simulink model "ctrl_PF"  (R2022b)
settings: Solver=FixedStepAuto  StartTime=0.0  StopTime=Tf  FixedStep=0.05  RelTol=1e-3
StopFcn:
  | save('testdata')
values from neighbouring files (symbols this model uses):
  Ba_0 = [0 0 0 0 0 0]    [run.m]    (also in testdata.mat)
  Bb = 4418825.3321    [testdata.mat]
  Bv_0 = [-5.14444 0 0 0 0 0]    [run.m]    (also in testdata.mat)
  Bx_0 = [-Cp(1,1) -Cp(2,1) Cp(3,1) 0 0 -pi]    [run.m]    (also in testdata.mat = [7.34788079488e-14 -400 -100 0 0 -3.14159265359])
  Cp = [x;y;z]    [run.m]    (also in testdata.mat = [-7.34788079488e-14 400 -100 -24.1026674607 399.273166418 -1)
  Cp_prime = Cp*Diff    [run.m]    (also in testdata.mat = [-4.77232815721 -0.143913049279 0 -4.75515990164 -0.42831409)
  d = 50    [run.m]    (also in testdata.mat)
  dA_BP1 = [0.00388591051125 0.00354364911083 0.00553040741788 0.00502167988714 0.0078585088908 0.00748424955325 0.0119232766011 0.0109054787122 0.0168329706434 0.016985509009 0.0156802934897 0.014556760782 ... (616 elements, 616x1)]    [testdata.mat]
  dA_BP2 = [0.00388594063171 0.00354357191533 0.00553040491113 0.00502170939051 0.00785855989083 0.00748435285791 0.0119232653011 0.0109054419481 0.0168329955973 0.0169854794658 0.015680230324 0.0145567225609 ... (616 elements, 616x1)]    [testdata.mat]
  dA_Hull = [0.896301676511 0.898896720864 0.884294141897 0.886832830172 0.870887902011 0.873360353662 0.856223658523 0.858613244346 0.840314828191 0.842595287849 0.823129385532 0.8253007603 ... (2914 elements, 2914x1)]    [testdata.mat]
  dA_PH = [0.00917454029683 0.00917454029683 0.00646521761836 0.00644666811643 0.011728531678 0.0107683420972 0.0165186720105 0.0100399866209 0.0121147162203 0.00917369783051 0.00917369783051 0.00646462373197 ... (550 elements, 550x1)]    [testdata.mat]
  dA_Sail = [0.08073747293 0.0655437895785 0.0678199581962 0.211496702297 0.185444652254 0.10949647106 0.0763960001413 0.0735864235671 0.0440728222699 0.281106392154 0.32735958292 0.104041938486 ... (564 elements, 564x1)]    [testdata.mat]
  dA_SProot = [0.0225345452169 0.0247277274893 0.0225345452169 0.0480467976325 0.0166447079844 0.0410754287554 0.0247277274893 0.0480467976325 0.0468898715351 0.0839833312794 0.0166447079844 0.0255016718 ... (904 elements, 904x1)]    [testdata.mat]
  dA_X1a = [0.0149621011817 0.0166706156701 0.0341149781095 0.0355915100668 0.0512235531199 0.0489176133683 0.0604458424392 0.0503279152264 0.0577124835488 0.0401555322121 0.044833653096 0.0251568218541 ... (200 elements, 200x1)]    [testdata.mat]
  dA_X1b = [0.0149621011817 0.0166706156701 0.0341149781095 0.0355915100668 0.0512235531199 0.0489176133683 0.0604458424392 0.0503279152264 0.0577124835488 0.0401555322121 0.044833653096 0.0251568218541 ... (200 elements, 200x1)]    [testdata.mat]
  dA_X2a = [0.0149620639393 0.0166705502855 0.0341150948266 0.0355913495849 0.051223110376 0.0489180393921 0.0604458270347 0.0503275686692 0.0577128112225 0.0401556683139 0.0448334591683 0.0251566482124 ... (200 elements, 200x1)]    [testdata.mat]
  dA_X2b = [0.0149620639393 0.0166705502855 0.0341150948266 0.0355913495849 0.051223110376 0.0489180393921 0.0604458270347 0.0503275686692 0.0577128112225 0.0401556683139 0.0448334591683 0.0251566482124 ... (200 elements, 200x1)]    [testdata.mat]
  dA_X3a = [0.0149621011817 0.0166706156701 0.0341149781095 0.0355915100668 0.0512235531199 0.0489176133683 0.0604458424392 0.0503279152264 0.0577124835488 0.0401555322121 0.044833653096 0.0251568218541 ... (200 elements, 200x1)]    [testdata.mat]
  dA_X3b = [0.0149621011817 0.0166706156701 0.0341149781095 0.0355915100668 0.0512235531199 0.0489176133683 0.0604458424392 0.0503279152264 0.0577124835488 0.0401555322121 0.044833653096 0.0251568218541 ... (200 elements, 200x1)]    [testdata.mat]
  dA_X4a = [0.0149621011817 0.0166706156701 0.0341149781095 0.0355915100668 0.0512235531199 0.0489176133683 0.0604458424392 0.0503279152264 0.0577124835488 0.0401555322121 0.044833653096 0.0251568218541 ... (200 elements, 200x1)]    [testdata.mat]
  dA_X4b = [0.0149621011817 0.0166706156701 0.0341149781095 0.0355915100668 0.0512235531199 0.0489176133683 0.0604458424392 0.0503279152264 0.0577124835488 0.0401555322121 0.044833653096 0.0251568218541 ... (200 elements, 200x1)]    [testdata.mat]
  Ixx = 52300000    [testdata.mat]
  Ixy = 0    [testdata.mat]
  Ixz = 0    [testdata.mat]
  Iyy = 1375000000    [testdata.mat]
  Iyz = 0    [testdata.mat]
  Izz = 1367000000    [testdata.mat]
  Ky = 1    [run.m]    (also in testdata.mat)
  Mb = 4418825.3321    [testdata.mat]
  n_BP1 = [-0.7747315 -0.03638153 -0.4095958 0 -0.1221389 0 -0.01670914 0 0.005209626 0 0.03404154 0 ... (1848 elements, 616x3)]    [testdata.mat]
  n_BP2 = [-0.774731517 -0.0363815315 -0.409595788 0 -0.122138903 0 -0.0167091396 0 0.00520962616 0 0.0340415388 0 ... (1848 elements, 616x3)]    [testdata.mat]
  n_Hull = [-3.334458e-05 -1.700098e-14 -3.354233e-05 -1.686235e-14 -3.289162e-05 -1.685701e-14 -3.291391e-05 -1.698144e-14 -3.338145e-05 -1.688959e-14 -3.29289e-05 -1.682536e-14 ... (8742 elements, 2914x3)]    [testdata.mat]
  n_PH = [0 0 0.01711651 0.01711627 0.2676807 0.2676804 0.7675173 0.7675174 0.9857236 0 0 0.01711456 ... (1650 elements, 550x3)]    [testdata.mat]
  n_Sail = [-0.05126832 -0.05168081 -0.0485872 -0.03288998 -0.03203588 -0.04435105 -0.04335441 -0.04419429 -0.05169604 0.01094904 0.01649325 -0.03825178 ... (1692 elements, 564x3)]    [testdata.mat]
  n_SProot = [-0.7837688 -0.7969784 -0.7837688 -0.79448 -0.280412 -0.3378876 -0.7969784 -0.79448 -0.7910827 -0.3483897 -0.280412 -0.2790298 ... (2712 elements, 904x3)]    [testdata.mat]
  n_X2a = [-0.283297986 -0.283136904 -0.283195704 -0.28313759 -0.2831586 -0.283137113 -0.28313911 -0.283136606 -0.283121586 -0.283136815 -0.283108413 -0.283138901 ... (600 elements, 200x3)]    [testdata.mat]
  n_X2b = [-0.283297986 -0.283136904 -0.283195704 -0.28313759 -0.2831586 -0.283137113 -0.28313911 -0.283136606 -0.283121586 -0.283136815 -0.283108413 -0.283138901 ... (600 elements, 200x3)]    [testdata.mat]
  n_X3a = [-0.283298 -0.2831369 -0.2831957 -0.2831376 -0.2831586 -0.2831371 -0.2831391 -0.2831366 -0.2831216 -0.2831368 -0.2831084 -0.2831389 ... (600 elements, 200x3)]    [testdata.mat]
  n_X4a = [-0.283298 -0.2831369 -0.2831957 -0.2831376 -0.2831586 -0.2831371 -0.2831391 -0.2831366 -0.2831216 -0.2831368 -0.2831084 -0.2831389 ... (600 elements, 200x3)]    [testdata.mat]
  n_X4b = [-0.283298 -0.2831369 -0.2831957 -0.2831376 -0.2831586 -0.2831371 -0.2831391 -0.2831366 -0.2831216 -0.2831368 -0.2831084 -0.2831389 ... (600 elements, 200x3)]    [testdata.mat]
  nt_BP1 = 616    [testdata.mat]
  nt_BP2 = 616    [testdata.mat]
  nt_Hull = 2914    [testdata.mat]
  nt_PH = 550    [testdata.mat]
  nt_Sail = 564    [testdata.mat]
  nt_SProot = 904    [testdata.mat]
  nt_X1a = 200    [testdata.mat]
  nt_X1b = 200    [testdata.mat]
  nt_X2a = 200    [testdata.mat]
  nt_X2b = 200    [testdata.mat]
  nt_X3a = 200    [testdata.mat]
  nt_X3b = 200    [testdata.mat]
  nt_X4a = 200    [testdata.mat]
  nt_X4b = 200    [testdata.mat]
  Seastate = 0    [run.m]    (also in testdata.mat)
  Tf = 500    [run.m]    (also in testdata.mat)
  v_ref = Bv_0(1)    [run.m]    (also in testdata.mat = -5.14444)
  vt1_BP1 = [-11.0524049722 -10.9924120522 -10.9924120522 -10.8819663922 -10.8819663922 -10.7297166322 -10.7297166322 -10.5070632922 -10.5070632922 -10.1807245522 -10.1807245522 -9.8815181122 ... (1848 elements, 616x3)]    [testdata.mat]
  vt1_BP2 = [-11.0524048318 -10.9924111396 -10.9924111396 -10.8819658306 -10.8819658306 -10.7297157898 -10.7297157898 -10.5070637134 -10.5070637134 -10.1807238502 -10.1807238502 -9.8815188844 ... (1848 elements, 616x3)]    [testdata.mat]
  vt1_Hull = [3.5122487678 3.7304022878 5.2621803278 5.4863499878 6.9866994878 7.2167238278 8.6832650078 8.9189474678 10.3493567078 10.5904445678 11.9823842078 12.2286247478 ... (8742 elements, 2914x3)]    [testdata.mat]
  vt1_PH = [37.3342788278 37.3342788278 37.4268866678 37.4268866678 37.5892452278 37.5892452278 37.7549453078 37.7549453078 37.8074619278 37.3342788278 37.3342788278 37.4268866678 ... (1650 elements, 550x3)]    [testdata.mat]
  vt1_Sail = [-12.4909433722 -12.1578443722 -12.0399645322 -11.2138368922 -10.6240515922 -11.5111900522 -11.9364967522 -11.6561249722 -12.4909433722 -7.5732648922 -6.8453119522 -11.1890071522 ... (1692 elements, 564x3)]    [testdata.mat]
  vt1_SProot = [29.2099766678 29.1371231078 29.0494854278 29.2099766678 29.2862630078 29.4526510478 29.0494854278 29.1261368078 29.3369263478 29.5706712878 29.0494854278 29.3857364078 ... (2712 elements, 904x3)]    [testdata.mat]
  vt1_X1a = [29.3961751478 29.4776282078 29.4776282078 29.7060309278 29.7060309278 30.0693861278 30.0693861278 30.5458756478 30.5458756478 31.0830460478 31.0830460478 31.6023926678 ... (600 elements, 200x3)]    [testdata.mat]
  vt1_X1b = [29.6638337078 29.6638337078 29.9620713878 29.9620713878 30.3181187678 30.3181187678 30.7116389078 30.7116389078 31.1104380878 31.1104380878 31.4810519678 31.4810519678 ... (600 elements, 200x3)]    [testdata.mat]
  vt1_X2a = [29.3961767624 29.4776272952 29.4776272952 29.7060326828 29.7060326828 30.0693842324 30.0693842324 30.5458736822 30.5458736822 31.083047171 31.083047171 31.6023916148 ... (600 elements, 200x3)]    [testdata.mat]
  vt1_X2b = [29.6638345502 29.6638345502 29.9620708964 29.9620708964 30.3181168022 30.3181168022 30.7116409436 30.7116409436 31.1104372454 31.1104372454 31.4810526698 31.4810526698 ... (600 elements, 200x3)]    [testdata.mat]
  vt1_X3a = [29.3961751478 29.4776282078 29.4776282078 29.7060309278 29.7060309278 30.0693861278 30.0693861278 30.5458756478 30.5458756478 31.0830460478 31.0830460478 31.6023926678 ... (600 elements, 200x3)]    [testdata.mat]
  vt1_X3b = [29.6638337078 29.6638337078 29.9620713878 29.9620713878 30.3181187678 30.3181187678 30.7116389078 30.7116389078 31.1104380878 31.1104380878 31.4810519678 31.4810519678 ... (600 elements, 200x3)]    [testdata.mat]
  vt1_X4a = [29.6638337078 29.6638337078 29.9620713878 29.9620713878 30.3181187678 30.3181187678 30.7116389078 30.7116389078 31.1104380878 31.1104380878 31.4810519678 31.4810519678 ... (600 elements, 200x3)]    [testdata.mat]
  vt1_X4b = [29.3961751478 29.4776282078 29.4776282078 29.7060309278 29.7060309278 30.0693861278 30.0693861278 30.5458756478 30.5458756478 31.0830460478 31.0830460478 31.6023926678 ... (600 elements, 200x3)]    [testdata.mat]
  vt2_BP1 = [-10.9924120522 -10.9494777322 -10.8819663922 -10.8505308322 -10.7297166322 -10.7112259522 -10.5070632922 -10.4997203722 -10.1807245522 -10.1757543922 -9.8815181122 -9.8813004922 ... (1848 elements, 616x3)]    [testdata.mat]
  vt2_BP2 = [-11.0294626294 -11.0294626294 -10.9494786448 -10.9494786448 -10.8505316746 -10.8505316746 -10.7112256012 -10.7112256012 -10.499720302 -10.499720302 -10.1757550942 -10.1757550942 ... (1848 elements, 616x3)]    [testdata.mat]
  vt2_Hull = [1.9517168078 1.9517168078 3.7304022878 3.7304022878 5.4863499878 5.4863499878 7.2167238278 7.2167238278 8.9189474678 8.9189474678 10.5904445678 10.5904445678 ... (8742 elements, 2914x3)]    [testdata.mat]
  vt2_PH = [37.2028433678 37.2028433678 37.3342788278 37.4268866678 37.4268866678 37.5892452278 37.5892452278 37.7549453078 37.7549453078 37.2028433678 37.2028433678 37.3342788278 ... (1650 elements, 550x3)]    [testdata.mat]
  vt2_Sail = [-12.0399645322 -12.0399645322 -11.9364967522 -10.7084881522 -10.7084881522 -12.0399645322 -12.0399645322 -11.9364967522 -12.3734566522 -7.7110323922 -7.7110323922 -11.6561249722 ... (1692 elements, 564x3)]    [testdata.mat]
  vt2_SProot = [29.0494854278 29.0494854278 29.2099766678 29.1261368078 29.0494854278 29.1371231078 29.1371231078 29.2099766678 29.1261368078 29.2099766678 29.2862630078 29.2862630078 ... (2712 elements, 904x3)]    [testdata.mat]
  vt2_X1a = [29.4776282078 29.9620713878 29.7060309278 30.3181187678 30.0693861278 30.7116389078 30.5458756478 31.1104380878 31.0830460478 31.4810519678 31.6023926678 31.7970362078 ... (600 elements, 200x3)]    [testdata.mat]
  vt2_X1b = [29.4776282078 29.9620713878 29.7060309278 30.3181187678 30.0693861278 30.7116389078 30.5458756478 31.1104380878 31.0830460478 31.4810519678 31.6023926678 31.7970362078 ... (600 elements, 200x3)]    [testdata.mat]
  vt2_X2a = [29.6638345502 29.6638345502 29.9620708964 29.9620708964 30.3181168022 30.3181168022 30.7116409436 30.7116409436 31.1104372454 31.1104372454 31.4810526698 31.4810526698 ... (600 elements, 200x3)]    [testdata.mat]
  vt2_X2b = [29.3961767624 29.4776272952 29.4776272952 29.7060326828 29.7060326828 30.0693842324 30.0693842324 30.5458736822 30.5458736822 31.083047171 31.083047171 31.6023916148 ... (600 elements, 200x3)]    [testdata.mat]
  vt2_X3a = [29.4776282078 29.9620713878 29.7060309278 30.3181187678 30.0693861278 30.7116389078 30.5458756478 31.1104380878 31.0830460478 31.4810519678 31.6023926678 31.7970362078 ... (600 elements, 200x3)]    [testdata.mat]
  vt2_X3b = [29.4776282078 29.9620713878 29.7060309278 30.3181187678 30.0693861278 30.7116389078 30.5458756478 31.1104380878 31.0830460478 31.4810519678 31.6023926678 31.7970362078 ... (600 elements, 200x3)]    [testdata.mat]
  vt2_X4a = [29.4776282078 29.9620713878 29.7060309278 30.3181187678 30.0693861278 30.7116389078 30.5458756478 31.1104380878 31.0830460478 31.4810519678 31.6023926678 31.7970362078 ... (600 elements, 200x3)]    [testdata.mat]
  vt2_X4b = [29.4776282078 29.9620713878 29.7060309278 30.3181187678 30.0693861278 30.7116389078 30.5458756478 31.1104380878 31.0830460478 31.4810519678 31.6023926678 31.7970362078 ... (600 elements, 200x3)]    [testdata.mat]
  vt3_BP1 = [-11.0294636122 -11.0294636122 -10.9494777322 -10.9494777322 -10.8505308322 -10.8505308322 -10.7112259522 -10.7112259522 -10.4997203722 -10.4997203722 -10.1757543922 -10.1757543922 ... (1848 elements, 616x3)]    [testdata.mat]
  vt3_BP2 = [-10.9924111396 -10.9494786448 -10.8819658306 -10.8505316746 -10.7297157898 -10.7112256012 -10.5070637134 -10.499720302 -10.1807238502 -10.1757550942 -9.8815188844 -9.8813013346 ... (1848 elements, 616x3)]    [testdata.mat]
  vt3_Hull = [1.7397198278 3.5122487678 3.5122487678 5.2621803278 5.2621803278 6.9866994878 6.9866994878 8.6832650078 8.6832650078 10.3493567078 10.3493567078 11.9823842078 ... (8742 elements, 2914x3)]    [testdata.mat]
  vt3_PH = [37.2028433678 37.3342788278 37.3342788278 37.3342788278 37.4268866678 37.4268866678 37.5892452278 37.5892452278 37.7549453078 37.2028433678 37.3342788278 37.3342788278 ... (1650 elements, 550x3)]    [testdata.mat]
  vt3_Sail = [-12.3734566522 -12.4909433722 -12.3734566522 -11.5111900522 -11.2138368922 -11.7698559922 -11.5111900522 -11.5111900522 -12.1578443722 -8.3109054322 -7.5732648922 -11.5111900522 ... (1692 elements, 564x3)]    [testdata.mat]
  vt3_SProot = [29.1261368078 29.2099766678 29.1261368078 29.3369263478 29.1371231078 29.2099766678 29.2099766678 29.3369263478 29.2548344678 29.3369263478 29.1371231078 29.1371231078 ... (2712 elements, 904x3)]    [testdata.mat]
  vt3_X1a = [29.6638337078 29.6638337078 29.9620713878 29.9620713878 30.3181187678 30.3181187678 30.7116389078 30.7116389078 31.1104380878 31.1104380878 31.4810519678 31.4810519678 ... (600 elements, 200x3)]    [testdata.mat]
  vt3_X1b = [29.3961751478 29.4776282078 29.4776282078 29.7060309278 29.7060309278 30.0693861278 30.0693861278 30.5458756478 30.5458756478 31.0830460478 31.0830460478 31.6023926678 ... (600 elements, 200x3)]    [testdata.mat]
  vt3_X2a = [29.4776272952 29.9620708964 29.7060326828 30.3181168022 30.0693842324 30.7116409436 30.5458736822 31.1104372454 31.083047171 31.4810526698 31.6023916148 31.7970343826 ... (600 elements, 200x3)]    [testdata.mat]
  vt3_X2b = [29.4776272952 29.9620708964 29.7060326828 30.3181168022 30.0693842324 30.7116409436 30.5458736822 31.1104372454 31.083047171 31.4810526698 31.6023916148 31.7970343826 ... (600 elements, 200x3)]    [testdata.mat]
  vt3_X3a = [29.6638337078 29.6638337078 29.9620713878 29.9620713878 30.3181187678 30.3181187678 30.7116389078 30.7116389078 31.1104380878 31.1104380878 31.4810519678 31.4810519678 ... (600 elements, 200x3)]    [testdata.mat]
  vt3_X3b = [29.3961751478 29.4776282078 29.4776282078 29.7060309278 29.7060309278 30.0693861278 30.0693861278 30.5458756478 30.5458756478 31.0830460478 31.0830460478 31.6023926678 ... (600 elements, 200x3)]    [testdata.mat]
  vt3_X4a = [29.3961751478 29.4776282078 29.4776282078 29.7060309278 29.7060309278 30.0693861278 30.0693861278 30.5458756478 30.5458756478 31.0830460478 31.0830460478 31.6023926678 ... (600 elements, 200x3)]    [testdata.mat]
  vt3_X4b = [29.6638337078 29.6638337078 29.9620713878 29.9620713878 30.3181187678 30.3181187678 30.7116389078 30.7116389078 31.1104380878 31.1104380878 31.4810519678 31.4810519678 ... (600 elements, 200x3)]    [testdata.mat]
  Xb = 0    [testdata.mat]
  Xcg = [32.3287332922 0 0]    [testdata.mat]
  Xg = 0    [testdata.mat]
  Yb = 0    [testdata.mat]
  Yg = 0    [testdata.mat]
  Zb = 0.4406    [testdata.mat]
  Zg = 0    [testdata.mat]
undefined symbols (not defined in the file or in its folder): Cpv
libraries: simulink x8, sharedtransform x2, dspmathops x2
(part 1 of 8)
settings Model: Creator=yagkim  LastModifiedBy=maclin
settings SolverCC: AlgebraicLoopSolver=TrustRegion
settings DebuggingCC: UnconnectedInputMsg=warning  UnconnectedOutputMsg=warning  UnconnectedLineMsg=warning  SFMachineParentedDataDiag=warning  ArithmeticOperatorsInVariantConditions=warning
settings ModelReferenceCC: EnableRefExpFcnMdlSchedulingChecks=on
settings SFSimCC: CustomCodeUndefinedFunction=UseInterfaceOnly
settings RTWCC: DLArmComputeVersion=19.05

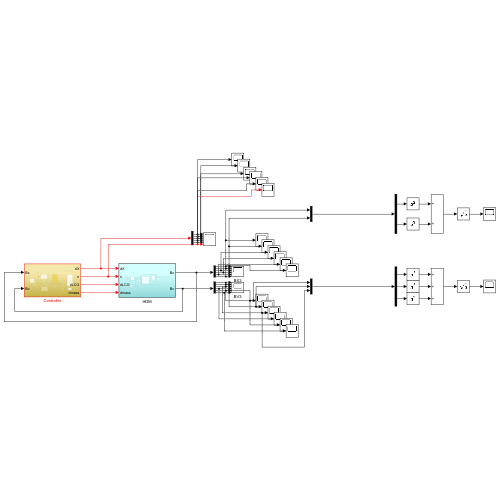
[thumbnail: Simulink's stored preview of the top-level diagram]
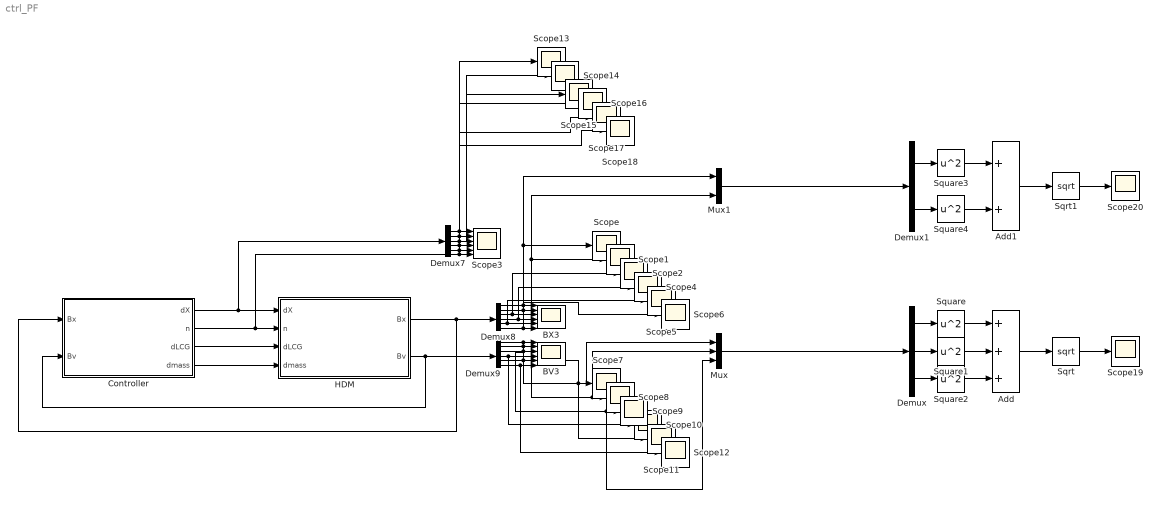
== system ctrl_PF ==
  Add : Sum  Inputs=+++
  Add1 : Sum
  BV3 : Scope  NumInputPorts=6
  BX3 : Scope  NumInputPorts=6
  Controller : Subsystem
  Demux : Demux  Outputs=3
  Demux1 : Demux  Outputs=2
  Demux7 : Demux  Outputs=5
  Demux8 : Demux  Outputs=6
  Demux9 : Demux  Outputs=6
  HDM : Subsystem
  Mux : Mux  Inputs=3
  Mux1 : Mux  Inputs=2
  Scope{,1..2,4..20} (20 alike) : Scope
  Scope3 : Scope  NumInputPorts=6
  Sqrt : Sqrt
  Sqrt1 : Sqrt
  Square{,1..4} (5 alike) : Math  Operator=square
  wires:
  Demux7/1 -> Scope13/1, Scope3/1
  Demux7/5 -> Scope17/1, Scope3/5
  Demux7/4 -> Scope16/1, Scope3/4
  Demux7/3 -> Scope15/1, Scope3/3
  Demux7/2 -> Scope14/1, Scope3/2
  Controller/4(dmass) -> HDM/4(dmass)
  Controller/3(dLCG) -> HDM/3(dLCG)
  Controller/1(dX) -> HDM/1(dX), Demux7/1
  Controller/2(n) -> HDM/2(n), Scope18/1, Scope3/6
  Demux8/1 -> Scope/1, Mux1/1, BX3/1
  Demux8/2 -> Mux1/2, Scope1/1, BX3/2
  Demux9/3 -> Mux/3, Scope9/1, BV3/3
  Demux8/3 -> BX3/3, Scope2/1
  Demux9/1 -> Mux/1, Scope7/1, BV3/1
  Demux8/4 -> BX3/4, Scope4/1
  Demux9/5 -> Scope11/1, BV3/5
  Demux8/6 -> Scope6/1, BX3/6
  Demux9/2 -> Mux/2, Scope8/1, BV3/2
  Demux8/5 -> BX3/5, Scope5/1
  Demux9/6 -> Scope12/1, BV3/6
  HDM/2(Bv) -> Demux9/1, Controller/2(Bv)
  Demux9/4 -> BV3/4, Scope10/1
  HDM/1(Bx) -> Demux8/1, Controller/1(Bx)
  Demux/2 -> Square1/1
  Square/1 -> Add/1
  Square1/1 -> Add/2
  Square2/1 -> Add/3
  Demux/3 -> Square2/1
  Mux/1 -> Demux/1
  Sqrt/1 -> Scope19/1
  Demux/1 -> Square/1
  Add/1 -> Sqrt/1
  Square4/1 -> Add1/2
  Demux1/2 -> Square4/1
  Mux1/1 -> Demux1/1
  Sqrt1/1 -> Scope20/1
  Add1/1 -> Sqrt1/1
  Square3/1 -> Add1/1
  Demux1/1 -> Square3/1

== system ctrl_PF/Controller ==
  Bx : Inport
  Bv : Inport  Port=2
  Constant : Constant  Value=-v_ref
  Constant1 : Constant  Value=0
  Constant2 : Constant  Value=Tf
  Constant3 : Constant  Value=[-1 0 0 0 0 0; 0 -1 0 0 0 0; 0 0 1 0 0 0; 0 0 0 1 0 0; 0 0 0 0 1 0; 0 0 0 0 0 1]
  Display : Display
  FF velocity ctrl : MATLAB Function  TreatAsAtomicUnit=on
  GreaterThan : RelationalOperator  OutDataTypeStr=boolean  RndMeth=Simplest  InputSameDT=off
  MATLAB Function1 : MATLAB Function  Commented=on  TreatAsAtomicUnit=on
  MATLAB Function2 : MATLAB Function  TreatAsAtomicUnit=on
  Marin PID : MATLAB Function  TreatAsAtomicUnit=on
  Matrix Multiply : Product  Multiplication=Matrix(*)
  Matrix Multiply1 : Product  Multiplication=Matrix(*)
  Scope : Scope
  Scope1 : Scope
  Scope2 : Scope
  Selector1 : Selector  InputPortWidth=6  IndexOptions=Index vector (dialog)  Indices=[1 2 3]  OutputSizes=1
  Selector2 : Selector  InputPortWidth=6  IndexOptions=Index vector (dialog)  Indices=[1]  OutputSizes=1
  Stop Simulation : Stop
  Subsystem1 : Subsystem
  dX : Outport
  n : Outport  Port=2
  dLCG : Outport  Port=3
  dmass : Outport  Port=4
  wires:
  Subsystem1/1(z_d) -> Marin PID/1(z_ref)
  FF velocity ctrl/1(n) -> Scope2/1, n/1
  Marin PID/1(dX) -> dX/1
  Constant1/1 -> dLCG/1, dmass/1
  MATLAB Function2/1(pd) -> Scope1/1, Subsystem1/1(pd(y))
  MATLAB Function2/2(pdp) -> Subsystem1/2(pd(y)')
  Subsystem1/2(psi_d) -> Marin PID/2(psi_ref)
  Selector1/1 -> Subsystem1/3(p)
  Subsystem1/3(gamma) -> GreaterThan/1, MATLAB Function2/1(gamma), MATLAB Function1/1(gamma)
  GreaterThan/1 -> Stop Simulation/1
  Constant2/1 -> Display/1, GreaterThan/2
  MATLAB Function1/1(v) -> Scope/1
  Selector2/1 -> Subsystem1/4(vel)
  Constant/1 -> FF velocity ctrl/1(v_ref)
  Bv/1 -> Matrix Multiply/2
  Matrix Multiply/1 -> Marin PID/3(Bv), Selector2/1
  Constant3/1 -> Matrix Multiply/1, Matrix Multiply1/1
  Bx/1 -> Matrix Multiply1/2
  Matrix Multiply1/1 -> Marin PID/4(Bx), Selector1/1

== system ctrl_PF/HDM ==
  dX : Inport
  n : Inport  Port=2
  dLCG : Inport  Port=3
  dmass : Inport  Port=4
  Constant1 : Constant  Value=Seastate
  HDM B3 : Subsystem  InitFcn='main'
  Integration and Coord. Transfrom : Subsystem
  Scope : Scope
  Scope1 : Scope
  actuator saturation : Subsystem
  Bx : Outport
  Bv : Outport  Port=2
  wires:
  actuator saturation/4(dmass (kg)) -> HDM B3/4(dmass), Scope1/1
  actuator saturation/3(dLCG (m)) -> HDM B3/3(dLCG)
  actuator saturation/2(n) -> HDM B3/2(n)
  actuator saturation/1(dX) -> HDM B3/1(dX CTRL)
  dmass/1 -> actuator saturation/4(dmass), Scope/1
  dLCG/1 -> actuator saturation/3(dLCG)
  n/1 -> actuator saturation/2("n ")
  dX/1 -> actuator saturation/1("dX ")
  Constant1/1 -> HDM B3/8(SeaState)
  HDM B3/1(F_hyd) -> Integration and Coord. Transfrom/2(F_hyd)
  Integration and Coord. Transfrom/3(Ba) -> HDM B3/7(Ba)
  Integration and Coord. Transfrom/1("Bx ") -> HDM B3/5(Bx), Integration and Coord. Transfrom/1(Bx), Bx/1
  Integration and Coord. Transfrom/2(Bv) -> HDM B3/6(Bv), Bv/1

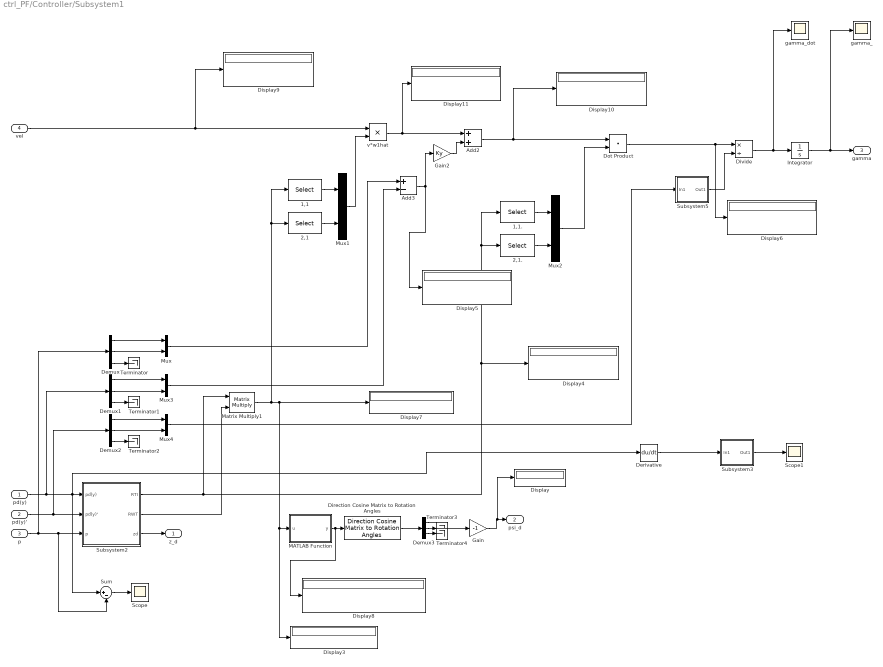
== system ctrl_PF/Controller/Subsystem1 ==
  pd(y) : Inport
  pd(y)' : Inport  Port=2
  p : Inport  Port=3
  vel : Inport  Port=4
  1,1 : Selector  NumberOfDimensions=2  InputPortWidth=3  IndexOptions=Index vector (dialog),Index vector (dialog)  Indices=1,1  OutputSizes=1,1
  1,1. : Selector  NumberOfDimensions=2  InputPortWidth=3  IndexOptions=Index vector (dialog),Index vector (dialog)  Indices=1,1  OutputSizes=1,1
  2,1 : Selector  NumberOfDimensions=2  InputPortWidth=3  IndexOptions=Index vector (dialog),Index vector (dialog)  Indices=2,1  OutputSizes=1,1
  2,1. : Selector  NumberOfDimensions=2  InputPortWidth=3  IndexOptions=Index vector (dialog),Index vector (dialog)  Indices=2,1  OutputSizes=1,1
  Add2 : Sum
  Add3 : Sum  Inputs=+-
  Demux{,1..3} (4 alike) : Demux  Outputs=3
  Derivative : Derivative
  Direction Cosine Matrix to Rotation Angles : sharedtransform/Direction Cosine Matrix to Rotation Angles  rotationOrder=ZYX  aMode=aMode  action=None  tolerance=eps(2)
      settings: LibrarySourceBlock=|
      | aerolibtransform2/Direction Cosine Matrix
      | to Rotation Angles
  Display{,3..11} (10 alike) : Display
  Divide : Product  Inputs=*/
  Dot Product : DotProduct  OutDataTypeStr=Inherit: Inherit via internal rule
  Gain : Gain  Gain=-1
  Gain2 : Gain  Gain=Ky
  Integrator : Integrator
  MATLAB Function : MATLAB Function  TreatAsAtomicUnit=on
  Matrix Multiply1 : Product  Multiplication=Matrix(*)
  Mux{,1..4} (5 alike) : Mux  Inputs=2
  Scope : Scope
  Scope1 : Scope
  Subsystem2 : Subsystem
  Subsystem3 : Subsystem
  Subsystem5 : Subsystem
  Sum : Sum  Inputs=|+-
  Terminator{,1..4} (5 alike) : Terminator
  gamma_ : Scope
  gamma_dot : Scope
  v*w1hat : Product
  z_d : Outport
  psi_d : Outport  Port=2
  gamma : Outport  Port=3
  wires:
  pd(y)'/1 -> Demux2/1, Subsystem2/2(pd(y)')
  pd(y)/1 -> Derivative/1, Sum/1, Subsystem2/1(pd(y)), Demux1/1
  p/1 -> Sum/2, Subsystem2/3(p), Demux/1
  Subsystem2/1(RTI) -> Matrix Multiply1/1, 1,1./1, 2,1./1, Display4/1
  vel/1 -> Display9/1, v*w1hat/1
  v*w1hat/1 -> Display11/1, Add2/1
  Gain2/1 -> Add2/2
  Add3/1 -> Gain2/1, Display5/1
  Dot Product/1 -> Display6/1, Divide/1
  Subsystem5/1(Out1) -> Divide/2
  Divide/1 -> gamma_dot/1, Integrator/1
  2,1/1 -> Mux1/2
  1,1/1 -> Mux1/1
  Mux1/1 -> v*w1hat/2
  1,1./1 -> Mux2/1
  2,1./1 -> Mux2/2
  Mux2/1 -> Dot Product/2
  Integrator/1 -> gamma_/1, gamma/1
  Add2/1 -> Display10/1, Dot Product/1
  Subsystem2/3(zd) -> z_d/1
  Subsystem2/2(RWT) -> Matrix Multiply1/2
  Demux/1 -> Mux/1
  Demux/2 -> Mux/2
  Demux/3 -> Terminator/1
  Demux1/1 -> Mux3/1
  Demux1/2 -> Mux3/2
  Demux1/3 -> Terminator1/1
  Demux2/1 -> Mux4/1
  Demux2/2 -> Mux4/2
  Demux2/3 -> Terminator2/1
  Mux/1 -> Add3/1
  Mux3/1 -> Add3/2
  Mux4/1 -> Subsystem5/1(In1)
  Sum/1 -> Scope/1
  Derivative/1 -> Subsystem3/1(In1)
  Subsystem3/1(Out1) -> Scope1/1
  MATLAB Function/1(y) -> Display8/1, Direction Cosine Matrix to Rotation Angles/1
  Demux3/1 -> Gain/1
  Direction Cosine Matrix to Rotation Angles/1 -> Demux3/1
  Matrix Multiply1/1 -> Display7/1, MATLAB Function/1(u), Display3/1, 2,1/1, 1,1/1
  Demux3/2 -> Terminator3/1
  Demux3/3 -> Terminator4/1
  Gain/1 -> Display/1, psi_d/1

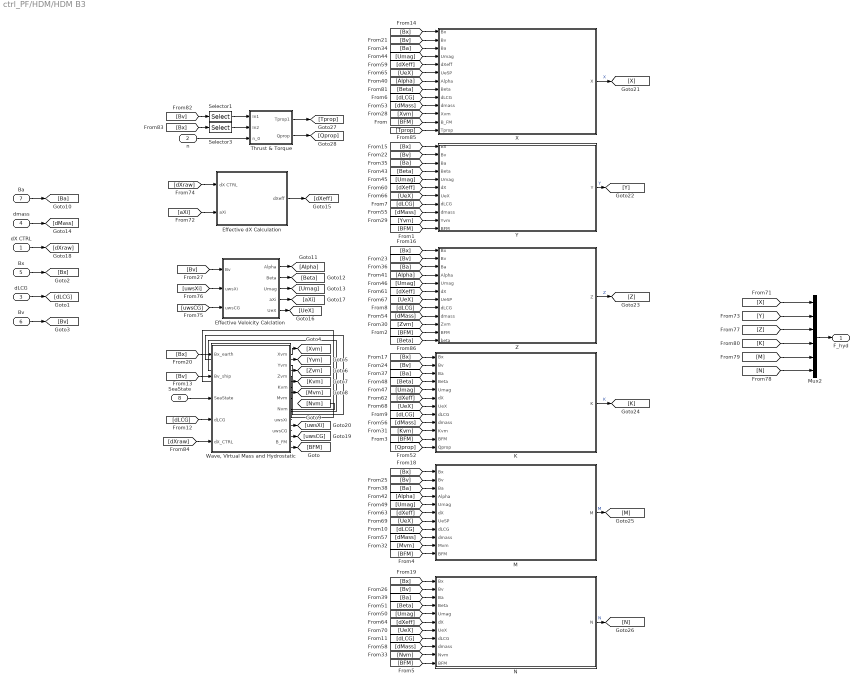
== system ctrl_PF/HDM/HDM B3 ==
  dX CTRL : Inport
  n : Inport  Port=2
  dLCG : Inport  Port=3
  dmass : Inport  Port=4
  Bx : Inport  Port=5
  Bv : Inport  Port=6
  Ba : Inport  Port=7
  SeaState : Inport  Port=8
  Effective Veloicity Calclation : Subsystem
  Effective dX Calculation : Subsystem
  K : Subsystem
  M : Subsystem
  Mux2 : Mux  Inputs=6
  N : Subsystem
  Selector1 : Selector  InputPortWidth=6  IndexOptions=Index vector (dialog)  Indices=1  OutputSizes=1
  Selector3 : Selector  InputPortWidth=6  IndexOptions=Index vector (dialog)  Indices=3  OutputSizes=1
  Thrust & Torque : Subsystem
  "Wave, Virtual Mass and Hydrostatic" : Subsystem
  X : Subsystem
  Y : Subsystem
  Z : Subsystem
  F_hyd : Outport  VectorParamsAs1DForOutWhenUnconnected=off
  wires:
  Z/1(Z) -> [Z]  "Z"
  [Beta] -> Z/12(beta)
  Thrust & Torque/2(Qprop) -> [Qprop]
  [Tprop] -> X/13(Tprop)
  Thrust & Torque/1(Tprop1) -> [Tprop]
  [Bx] -> Selector3/1
  Selector3/1 -> Thrust & Torque/2(In2)
  Selector1/1 -> Thrust & Torque/1(In1)
  [Bv] -> Selector1/1
  [Qprop] -> K/12(Qprop)
  [N] -> Mux2/6
  [M] -> Mux2/5
  [K] -> Mux2/4
  [Z] -> Mux2/3
  [Y] -> Mux2/2
  [X] -> Mux2/1
  [dXraw] -> "Wave, Virtual Mass and Hydrostatic"/5(dX_CTRL)
  [Beta] -> X/8(Beta)
  N/1(N) -> [N]  "N"
  M/1(M) -> [M]  "M"
  K/1(K) -> [K]  "K"
  Y/1(Y) -> [Y]  "Y"
  X/1(X) -> [X]  "X"
  [uwsXi] -> Effective Veloicity Calclation/2(uwsXi)
  "Wave, Virtual Mass and Hydrostatic"/7(uwsXi) -> [uwsXi]
  [uwsCG] -> Effective Veloicity Calclation/3(uwsCG)
  "Wave, Virtual Mass and Hydrostatic"/8(uwsCG) -> [uwsCG]
  [dXraw] -> Effective dX Calculation/1(dX CTRL)
  dX CTRL/1 -> [dXraw]
  [aXi] -> Effective dX Calculation/2(aXi)
  Effective Veloicity Calclation/4(aXi) -> [aXi]
  [UeX] -> N/7(UeX)
  [UeX] -> M/7(UeSP)
  [UeX] -> K/7(UeX)
  [UeX] -> Z/7(UeSP)
  [UeX] -> Y/7(UeX)
  [UeX] -> X/6(UeSP)
  Effective Veloicity Calclation/5(UeX) -> [UeX]
  [dXeff] -> N/6(dX)
  [dXeff] -> M/6(dX)
  [dXeff] -> K/6(dX)
  [dXeff] -> Z/6(dX)
  [dXeff] -> Y/6(dX)
  [dXeff] -> X/5(dXeff)
  [dMass] -> N/9(dmass)
  [dMass] -> M/9(dmass)
  [dMass] -> K/9(dmass)
  [dMass] -> Y/9(dmass)
  [dMass] -> Z/9(dmass)
  [dMass] -> X/10(dmass)
  dmass/1 -> [dMass]
  [Beta] -> N/4(Beta)
  [Umag] -> N/5(Umag)
  [Umag] -> M/5(Umag)
  [Beta] -> K/4(Beta)
  [Umag] -> K/5(Umag)
  [Umag] -> Z/5(Umag)
  [Umag] -> Y/5(Umag)
  [Umag] -> X/4(Umag)
  Effective Veloicity Calclation/3(Umag) -> [Umag]
  [Beta] -> Y/4(Beta)
  Effective Veloicity Calclation/2(Beta) -> [Beta]
  [Alpha] -> M/4(Alpha)
  [Alpha] -> Z/4(Alpha)
  [Alpha] -> X/7(Alpha)
  Effective Veloicity Calclation/1(Alpha) -> [Alpha]
  [Ba] -> N/3(Ba)
  [Ba] -> M/3(Ba)
  [Ba] -> K/3(Ba)
  [Ba] -> Z/3(Ba)
  [Ba] -> Y/3(Ba)
  [Ba] -> X/3(Ba)
  [Nvm] -> N/10(Nvm)
  [Mvm] -> M/10(Mvm)
  [Kvm] -> K/10(Kvm)
  [Bv] -> Z/2(Bv)
  [Zvm] -> Z/10(Zvm)
  [Yvm] -> Y/10(Yvm)
  [Xvm] -> X/11(Xvm)
  "Wave, Virtual Mass and Hydrostatic"/6(Nvm) -> [Nvm]
  "Wave, Virtual Mass and Hydrostatic"/5(Mvm) -> [Mvm]
  "Wave, Virtual Mass and Hydrostatic"/4(Kvm) -> [Kvm]
  "Wave, Virtual Mass and Hydrostatic"/3(Zvm) -> [Zvm]
  "Wave, Virtual Mass and Hydrostatic"/2(Yvm) -> [Yvm]
  "Wave, Virtual Mass and Hydrostatic"/1(Xvm) -> [Xvm]
  [Bv] -> Effective Veloicity Calclation/1(Bv)
  [Bv] -> N/2(Bv)
  [Bv] -> M/2(Bv)
  [Bv] -> K/2(Bv)
  [Bv] -> Y/2(Bv)
  [Bv] -> X/2(Bv)
  [Bv] -> "Wave, Virtual Mass and Hydrostatic"/2(Bv_ship)
  [Bx] -> "Wave, Virtual Mass and Hydrostatic"/1(Bx_earth)
  [Bx] -> N/1(Bx)
  [Bx] -> M/1(Bx)
  [Bx] -> K/1(Bx)
  [Bx] -> Z/1(Bx)
  [Bx] -> Y/1(Bx)
  [Bx] -> X/1(Bx)
  [dLCG] -> "Wave, Virtual Mass and Hydrostatic"/4(dLCG)
  [dLCG] -> N/8(dLCG)
  [dLCG] -> M/8(dLCG)
  [dLCG] -> K/8(dLCG)
  [dLCG] -> Z/8(dLCG)
  [dLCG] -> Y/8(dLCG)
  [dLCG] -> X/9(dLCG)
  [BFM] -> N/11(BFM)
  [BFM] -> M/11(BFM)
  [BFM] -> K/11(BFM)
  [BFM] -> Z/11(BFM)
  [BFM] -> Y/11(BFM)
  [BFM] -> X/12(B_FM)
  "Wave, Virtual Mass and Hydrostatic"/9(B_FM) -> [BFM]
  n/1 -> Thrust & Torque/3(n_0)
  SeaState/1 -> "Wave, Virtual Mass and Hydrostatic"/3(SeaState)
  Bv/1 -> [Bv]
  dLCG/1 -> [dLCG]
  Bx/1 -> [Bx]
  Ba/1 -> [Ba]
  Effective dX Calculation/1(dXeff) -> [dXeff]
  Mux2/1 -> F_hyd/1

== system ctrl_PF/HDM/Integration and Coord. Transfrom ==
  Bx : Inport
  F_hyd : Inport  Port=2
  Coordinate Transform : Subsystem
  Rigid Body Motion : Subsystem
  "Bx " : Outport
  Bv : Outport  Port=2
  Ba : Outport  Port=3
  wires:
  Bx/1 -> Rigid Body Motion/2(Bx)
  F_hyd/1 -> Rigid Body Motion/1(F_hyd)
  Rigid Body Motion/2(Ba) -> Ba/1
  Rigid Body Motion/1(Bv) -> Bv/1, Coordinate Transform/1(Bv)
  Coordinate Transform/1(X_earth) -> "Bx "/1

== system ctrl_PF/HDM/actuator saturation ==
  "dX " : Inport
  "n " : Inport  Port=2
  dLCG : Inport  Port=3
  dmass : Inport  Port=4
  " " : Subsystem
  "   " : Subsystem
  Subsystem1 : Subsystem
  Subsystem2 : Subsystem
  dX : Outport
  n : Outport  Port=2
  dLCG (m) : Outport  Port=3
  dmass (kg) : Outport  Port=4
  wires:
  "n "/1 -> "   "/1("n ")
  Subsystem2/1(dmass (kg)) -> dmass (kg)/1
  "dX "/1 -> " "/1("dX ")
  dmass/1 -> Subsystem2/1(dmass)
  Subsystem1/1(dLCG (m)) -> dLCG (m)/1
  dLCG/1 -> Subsystem1/1(dLCG)
  " "/1(dX) -> dX/1
  "   "/1(n) -> n/1

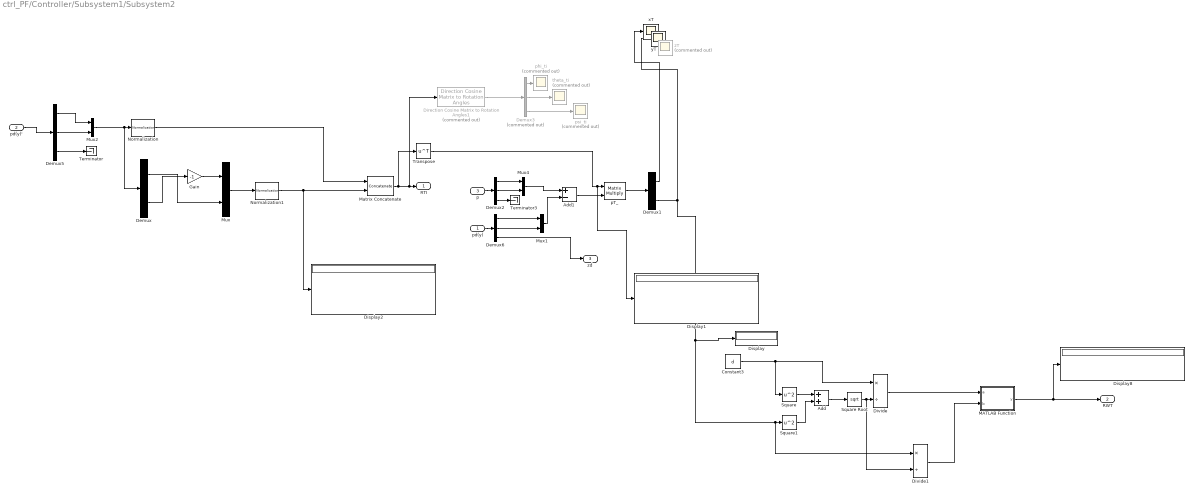
== system ctrl_PF/Controller/Subsystem1/Subsystem2 ==
  pd(y) : Inport
  pd(y)' : Inport  Port=2
  p : Inport  Port=3
  Add : Sum
  Add1 : Sum  Inputs=+-
  Constant3 : Constant  Value=d
  Demux : Demux  Outputs=2
  Demux1 : Demux  Outputs=2
  Demux2 : Demux  Outputs=3
  Demux3 : Demux  Commented=on  Outputs=3
  Demux5 : Demux  Outputs=3
  Demux6 : Demux  Outputs=3
  Direction Cosine Matrix to Rotation Angles1 : sharedtransform/Direction Cosine Matrix to Rotation Angles  Commented=on  rotationOrder=XYZ  aMode=aMode  action=None  tolerance=eps(2)
  Display{,1..2,8} (4 alike) : Display
  Divide : Product  Inputs=*/
  Divide1 : Product  Inputs=*/
  Gain : Gain  Gain=-1
  MATLAB Function : MATLAB Function  TreatAsAtomicUnit=on
  Matrix Concatenate : Concatenate  Mode=Multidimensional array  ConcatenateDimension=2
  Mux{,1..2,4} (4 alike) : Mux  Inputs=2
  Normalization : dspmathops/Normalization  NormType=2-norm  Bias=1e-10  NormOver=Each column  Dimension=1  roundingMode=Floor  overflowMode=off  accumDataTypeStr=Inherit: Same as product output  accumLastDataTypeStr=Inherit: Same as product output  outputDataTypeStr=Inherit: Same as product output  outputMin=[]  outputMax=[]  outputLastDataTypeStr=Inherit: Same as product output
  Normalization1 : dspmathops/Normalization  NormType=2-norm  Bias=1e-10  NormOver=Each column  Dimension=1  roundingMode=Floor  overflowMode=off  accumDataTypeStr=Inherit: Same as product output  accumLastDataTypeStr=Inherit: Same as product output  outputDataTypeStr=Inherit: Same as product output  outputMin=[]  outputMax=[]  outputLastDataTypeStr=Inherit: Same as product output
  Square : Math  Operator=square
  Square Root : Sqrt
  Square1 : Math  Operator=square
  Terminator : Terminator
  Terminator3 : Terminator
  Transpose : Math  Operator=transpose
  pT_ : Product  Multiplication=Matrix(*)
  phi_ti : Scope  Commented=on
  psi_ti : Scope  Commented=on
  theta_ti : Scope  Commented=on
  xT : Scope
  yT : Scope
  zT : Scope  Commented=on
  RTI : Outport
  RWT : Outport  Port=2
  zd : Outport  Port=3
  wires:
  Gain/1 -> Mux/1
  Demux/2 -> Gain/1
  Demux/1 -> Mux/2
  Mux/1 -> Normalization1/1
  Normalization/1 -> Matrix Concatenate/1
  Normalization1/1 -> Matrix Concatenate/2, Display2/1
  Matrix Concatenate/1 -> Direction Cosine Matrix to Rotation Angles1/1, RTI/1, Transpose/1
  Transpose/1 -> Display1/1, pT_/1
  Add1/1 -> pT_/2
  pT_/1 -> Demux1/1
  Demux1/2 -> yT/1, Display/1, Divide1/1, Square1/1
  Demux1/1 -> xT/1
  Direction Cosine Matrix to Rotation Angles1/1 -> Demux3/1
  Demux3/3 -> psi_ti/1
  Demux3/2 -> theta_ti/1
  Demux3/1 -> phi_ti/1
  Constant3/1 -> Square/1, Divide/1
  Square Root/1 -> Divide1/2, Divide/2
  Add/1 -> Square Root/1
  Square/1 -> Add/1
  Square1/1 -> Add/2
  Divide/1 -> MATLAB Function/1(a)
  Divide1/1 -> MATLAB Function/2(b)
  MATLAB Function/1(y) -> RWT/1, Display8/1
  Demux6/3 -> zd/1
  pd(y)'/1 -> Demux5/1
  Mux2/1 -> Demux/1, Normalization/1
  Demux5/1 -> Mux2/1
  Demux5/2 -> Mux2/2
  Demux5/3 -> Terminator/1
  Demux2/1 -> Mux4/1
  Demux2/3 -> Terminator3/1
  Demux2/2 -> Mux4/2
  Mux4/1 -> Add1/1
  p/1 -> Demux2/1
  Demux6/1 -> Mux1/1
  Demux6/2 -> Mux1/2
  pd(y)/1 -> Demux6/1
  Mux1/1 -> Add1/2

== system ctrl_PF/Controller/Subsystem1/Subsystem3 ==
  In1 : Inport
  Add : Sum  Inputs=+++
  Demux : Demux  Outputs=3
  Sqrt : Sqrt
  Square : Math  Operator=square
  Square1 : Math  Operator=square
  Square2 : Math  Operator=square
  Out1 : Outport
  wires:
  Sqrt/1 -> Out1/1
  Square1/1 -> Add/2
  Square/1 -> Add/1
  Add/1 -> Sqrt/1
  Demux/2 -> Square1/1
  Demux/1 -> Square/1
  In1/1 -> Demux/1
  Demux/3 -> Square2/1
  Square2/1 -> Add/3

== system ctrl_PF/Controller/Subsystem1/Subsystem5 ==
  In1 : Inport
  Add : Sum
  Demux : Demux  Outputs=2
  Sqrt : Sqrt
  Square : Math  Operator=square
  Square1 : Math  Operator=square
  Out1 : Outport
  wires:
  In1/1 -> Demux/1
  Demux/1 -> Square/1
  Demux/2 -> Square1/1
  Add/1 -> Sqrt/1
  Square/1 -> Add/1
  Square1/1 -> Add/2
  Sqrt/1 -> Out1/1

== system ctrl_PF/HDM/HDM B3/Effective Veloicity Calclation ==
  Bv : Inport
  uwsXi : Inport  Port=2
  uwsCG : Inport  Port=3
  Add{,1..4} (5 alike) : Sum
  Demux : Demux  Outputs=5
  Demux1 : Demux  Outputs=3
  MATLAB Function : MATLAB Function  TreatAsAtomicUnit=on
  MATLAB Function1 : MATLAB Function  TreatAsAtomicUnit=on
  MATLAB Function2 : MATLAB Function  TreatAsAtomicUnit=on
  X_SP1 : Constant  Value=[31.924; 3.861; -3.861;]
  X_SP2 : Constant  Value=[31.924; 3.861; 3.861;]
  X_SP3 : Constant  Value=[31.924; -3.861; 3.861;]
  X_SP4 : Constant  Value=[31.924; -3.861; -3.861;]
  X_XB : Constant  Value=[-10.465; 0; 9.732;]
  n1 : Constant  Value=[0; 1/sqrt(2); -1/sqrt(2);]
  n2 : Constant  Value=[0; 1/sqrt(2); 1/sqrt(2);]
  n3 : Constant  Value=[0; -1/sqrt(2); 1/sqrt(2);]
  n4 : Constant  Value=[0; -1/sqrt(2); -1/sqrt(2);]
  n5 : Constant  Value=[0; 1; 0;]
  nh : Constant  Value=[-1; 0; 0;]
  Alpha : Outport
  Beta : Outport  Port=2
  Umag : Outport  Port=3
  aXi : Outport  Port=4
  UeX : Outport  Port=5
  wires:
  uwsXi/1 -> Demux/1
  MATLAB Function/1(aX) -> aXi/1
  MATLAB Function2/1(alpha) -> Alpha/1
  uwsCG/1 -> Demux1/1
  Demux1/3 -> MATLAB Function2/4(wCG)
  Demux1/2 -> MATLAB Function2/3(vCG)
  Demux1/1 -> MATLAB Function2/2(uCG)
  MATLAB Function/2(UeX) -> UeX/1
  MATLAB Function2/3(Umag) -> Umag/1
  MATLAB Function2/2(beta) -> Beta/1
  MATLAB Function1/2(urX2) -> Add1/1
  MATLAB Function1/3(urX3) -> Add2/1
  MATLAB Function1/4(urX4) -> Add3/1
  MATLAB Function1/5(urXB) -> Add4/1
  Demux/5 -> Add4/2
  Demux/4 -> Add3/2
  Demux/3 -> Add2/2
  Demux/2 -> Add1/2
  Add4/1 -> MATLAB Function/11(urXB)
  Add3/1 -> MATLAB Function/10(urX4)
  Add2/1 -> MATLAB Function/9(urX3)
  Add1/1 -> MATLAB Function/8(urX2)
  Add/1 -> MATLAB Function/7(urX1)
  Demux/1 -> Add/2
  MATLAB Function1/1(urX1) -> Add/1
  n5/1 -> MATLAB Function/6(nB)
  X_SP1/1 -> MATLAB Function1/1(rX1)
  X_SP4/1 -> MATLAB Function1/4(rX4)
  X_SP3/1 -> MATLAB Function1/3(rX3)
  X_SP2/1 -> MATLAB Function1/2(rX2)
  X_XB/1 -> MATLAB Function1/5(rXB)
  n4/1 -> MATLAB Function/5(n4)
  n3/1 -> MATLAB Function/4(n3)
  n2/1 -> MATLAB Function/3(n2)
  n1/1 -> MATLAB Function/2(n1)
  nh/1 -> MATLAB Function/1(nh)
  Bv/1 -> MATLAB Function2/1(Bv), MATLAB Function1/6(U_ship)

== system ctrl_PF/HDM/HDM B3/Effective dX Calculation ==
  dX CTRL : Inport
  aXi : Inport  Port=2
  Add{,1..4} (5 alike) : Sum
  Demux : Demux  Outputs=5
  Demux1 : Demux  Outputs=5
  Mux6 : Mux  Inputs=5
  dXeff : Outport
  wires:
  Mux6/1 -> dXeff/1
  Demux1/5 -> Add4/2
  Demux1/4 -> Add3/2
  Demux1/3 -> Add2/2
  Demux1/2 -> Add1/2
  Demux1/1 -> Add/2
  Demux/5 -> Add4/1
  Demux/4 -> Add3/1
  Demux/3 -> Add2/1
  Demux/2 -> Add1/1
  Demux/1 -> Add/1
  Add4/1 -> Mux6/5
  Add3/1 -> Mux6/4
  Add2/1 -> Mux6/3
  Add1/1 -> Mux6/2
  Add/1 -> Mux6/1
  aXi/1 -> Demux1/1
  dX CTRL/1 -> Demux/1

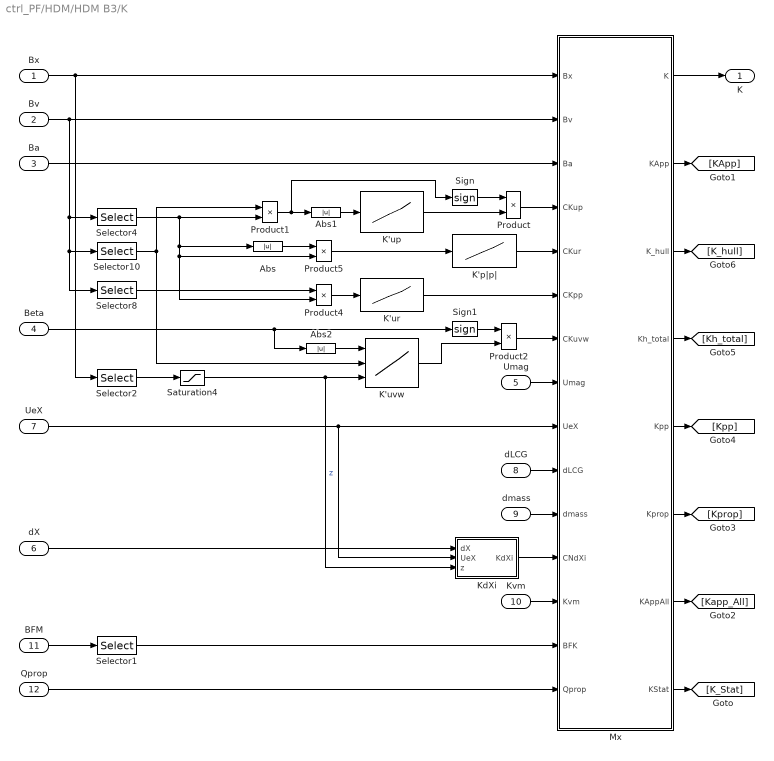
== system ctrl_PF/HDM/HDM B3/K ==
  Bx : Inport
  Bv : Inport  Port=2
  Ba : Inport  Port=3
  Beta : Inport  Port=4
  Umag : Inport  Port=5
  dX : Inport  Port=6
  UeX : Inport  Port=7
  dLCG : Inport  Port=8
  dmass : Inport  Port=9
  Kvm : Inport  Port=10
  BFM : Inport  Port=11
  Qprop : Inport  Port=12
  Abs : Abs  SaturateOnIntegerOverflow=off
  Abs1 : Abs  SaturateOnIntegerOverflow=off
  Abs2 : Abs  SaturateOnIntegerOverflow=off
  K'p|p| : Lookup_n-D  NumberOfTableDimensions=1  BreakpointsForDimension1=|  Table=|  InternalRulePriority=Speed  RndMeth=Simplest
      BreakpointsForDimension1=|
      | [-0.0015
      | -0.0012
      | -0.0009
      | -0.0006
      | -0.0003
      | -0.0001
      | 0.0001
      | 0.0003
      | 0.0006
      | 0.0009
      | 0.0012
      | 0.0015]
      Table=|
      | [-1.3011E-02
      | -1.6962E-02
      | -2.0682E-02
      | -3.1419E-02
      | -6.4407E-02
      | -1.9322E-01
      | 1.9322E-01
      | 6.4378E-02
      | 3.1944E-02
      | 2.1072E-02
      | 1.6415E-02
      | 1.3407E-02]
  K'up : Lookup_n-D  NumberOfTableDimensions=1  BreakpointsForDimension1=|  Table=|  InternalRulePriority=Speed  RndMeth=Simplest
      BreakpointsForDimension1=|
      | [0.03999989
      | 0.079999993
      | 0.11999963
      | 0.15999956]
      Table=|
      | [-4.0344E-04
      | -8.1402E-04
      | -1.2116E-03
      | -1.6125E-03]
  K'ur : Lookup_n-D  NumberOfTableDimensions=1  BreakpointsForDimension1=|  Table=|  InternalRulePriority=Speed  RndMeth=Simplest
      BreakpointsForDimension1=|
      | [-0.0015
      | -0.0012
      | -0.0009
      | -0.0006
      | -0.0003
      | -0.0001
      | 0.0001
      | 0.0003
      | 0.0006
      | 0.0009
      | 0.0012
      | 0.0015]
      Table=|
      | [-1.3011E-02
      | -1.6962E-02
      | -2.0682E-02
      | -3.1419E-02
      | -6.4407E-02
      | -1.9322E-01
      | 1.9322E-01
      | 6.4378E-02
      | 3.1944E-02
      | 2.1072E-02
      | 1.6415E-02
      | 1.3407E-02]
  K'uvw : Lookup_n-D  NumberOfTableDimensions=3  BreakpointsForDimension1=|  BreakpointsForDimension2=|  BreakpointsForDimension3=|  Table=|  InternalRulePriority=Speed  RndMeth=Simplest
      BreakpointsForDimension1=|
      | [0
      | 4
      | 8
      | 12]
      BreakpointsForDimension2=|
      | [-5.1444E+00
      | -3.0866E+00
      | -1.5433E+00
      | ]
      Table=|
      | reshape([0.0000000E+00
      | 1.5570290E-04
      | 3.7677829E-04
      | 6.0025374E-04
      | 0.0000000E+00
      | 1.5575678E-04
      | 3.8557685E-04
      | 6.0103850E-04
      | 0.0000000E+00
      | 1.7511088E-04
      | 3.8376789E-04
      | 6.0108480E-04
      | 0.0000000E+00
      | 1.9071552E-04
      | 4.0986649E-04
      | 6.4012030E-04
      | 0.0000000E+00
      | 1.8940622E-04
      | 4.0946931E-04
      | 6.3613461E-04
      | 0.0000000E+00
      | 1.8621071E-04
      | 4.0619654E-04
      | 7.0286379E-04
      | 0.0000000E+00
      | 2.0712189E-04
      | 4.4751988E-04
      | 7.0514631E-04
      | 0.0000000E+00
      | 1.9895751E-04
      | 4.3099356E-04
      | 6.6994571E-04
      | 0.0000000E+00
      | 1.9568554E-04
      | 4.2679977E-04
      | 6.6445067E-04
      | 0.0000000E+00
      | 2.4359563E-04
      | 5.3740096E-04
      | 8.5879902E-04
      | 0.0000000E+00
      | 2.0890025E-04
      | 4.5502130E-04
      | 7.1388224E-04
      | 0.0000000E+00
      | 2.0575072E-04
      | 4.5505766E-04
      | 7.0285206E-04],[4,3,4])
      BreakpointsForDimension3=|
      | [-35.0624 -18.3724 -15.3724 -13.8724
      | ]
      settings: InputPortMap=u0,u1,u2
  KdXi : Subsystem
  Mx : MATLAB Function  TreatAsAtomicUnit=on
  Product{,1..2,4..5} (5 alike) : Product
  Saturation4 : Saturate  UpperLimit=-13.8724  LowerLimit=-35.0624
  Selector1 : Selector  InputPortWidth=6  IndexOptions=Index vector (dialog)  Indices=4  OutputSizes=1
  Selector10 : Selector  InputPortWidth=6  IndexOptions=Index vector (dialog)  Indices=1  OutputSizes=1
  Selector2 : Selector  InputPortWidth=6  IndexOptions=Index vector (dialog)  Indices=3  OutputSizes=1
  Selector4 : Selector  InputPortWidth=6  IndexOptions=Index vector (dialog)  Indices=4  OutputSizes=1
  Selector8 : Selector  InputPortWidth=6  IndexOptions=Index vector (dialog)  Indices=2  OutputSizes=1
  Sign : Signum
  Sign1 : Signum
  K : Outport
  wires:
  Mx/3(K_hull) -> [K_hull]
  Mx/4(Kh_total) -> [Kh_total]
  Mx/5(Kpp) -> [Kpp]
  Mx/6(Kprop) -> [Kprop]
  Mx/7(KAppAll) -> [Kapp_All]
  Mx/2(KApp) -> [KApp]
  Qprop/1 -> Mx/15(Qprop)
  Kvm/1 -> Mx/13(Kvm)
  Saturation4/1 -> K'uvw/3, KdXi/3(z)  "z"
  K'p|p|/1 -> Mx/5(CKur)
  Product/1 -> Mx/4(CKup)
  Sign1/1 -> Product2/1
  Mx/8(KStat) -> [K_Stat]
  Mx/1(K) -> K/1
  Selector1/1 -> Mx/14(BFK)
  BFM/1 -> Selector1/1
  Abs2/1 -> K'uvw/1
  Product2/1 -> Mx/7(CKuvw)
  Sign/1 -> Product/1
  Abs1/1 -> K'up/1
  Product1/1 -> Abs1/1, Sign/1
  K'uvw/1 -> Product2/2
  Selector2/1 -> Saturation4/1
  KdXi/1(KdXi) -> Mx/12(CNdXi)
  K'ur/1 -> Mx/6(CKpp)
  Selector4/1 -> Product1/2, Abs/1, Product5/2, Product4/2
  Product5/1 -> K'p|p|/1
  Abs/1 -> Product5/1
  Selector8/1 -> Product4/1
  Product4/1 -> K'ur/1
  K'up/1 -> Product/2
  dX/1 -> KdXi/1(dX)
  dmass/1 -> Mx/11(dmass)
  dLCG/1 -> Mx/10(dLCG)
  Umag/1 -> Mx/8(Umag)
  Beta/1 -> Sign1/1, Abs2/1
  UeX/1 -> KdXi/2(UeX), Mx/9(UeX)
  Ba/1 -> Mx/3(Ba)
  Selector10/1 -> Product1/1, K'uvw/2
  Bx/1 -> Selector2/1, Mx/1(Bx)
  Bv/1 -> Mx/2(Bv), Selector4/1, Selector10/1, Selector8/1

== system ctrl_PF/HDM/HDM B3/M ==
  Bx : Inport
  Bv : Inport  Port=2
  Ba : Inport  Port=3
  Alpha : Inport  Port=4
  Umag : Inport  Port=5
  dX : Inport  Port=6
  UeSP : Inport  Port=7
  dLCG : Inport  Port=8
  dmass : Inport  Port=9
  Mvm : Inport  Port=10
  BFM : Inport  Port=11
  Abs : Abs  SaturateOnIntegerOverflow=off
  Gain : Gain  Gain=1.1
  Gain1 : Gain  Gain=1.3
  M'prop : Lookup_n-D  NumberOfTableDimensions=1  BreakpointsForDimension1=[-7.7166666 -5.1444444 -3.08666664]  Table=[-0.00022 -0.0002 -0.00015]  InternalRulePriority=Speed  RndMeth=Simplest
  M_uvwa : Lookup_n-D  NumberOfTableDimensions=3  BreakpointsForDimension1=|  BreakpointsForDimension2=|  BreakpointsForDimension3=|  Table=|  InternalRulePriority=Speed  RndMeth=Simplest
      BreakpointsForDimension1=|
      | [-12
      | -8
      | -4
      | 0
      | 4
      | 8
      | 12]
      BreakpointsForDimension2=|
      | [-5.1444E+00
      | -3.0866E+00
      | -1.5433E+00
      | ]
      Table=|
      | reshape([-2.40251E-03
      | -1.59538E-03
      | -8.21748E-04
      | -3.60182E-06
      | 8.13350E-04
      | 1.50586E-03
      | 2.39707E-03
      | -2.43392E-03
      | -1.61509E-03
      | -8.50748E-04
      | -3.60182E-06
      | 8.24271E-04
      | 1.51842E-03
      | 2.43805E-03
      | -2.45014E-03
      | -1.65711E-03
      | -9.11210E-04
      | -3.60182E-06
      | 8.61300E-04
      | 1.57459E-03
      | 2.42777E-03
      | -2.54380E-03
      | -1.68842E-03
      | -8.33041E-04
      | 2.23377E-05
      | 8.77717E-04
      | 1.73310E-03
      | 2.58847E-03
      | -2.63734E-03
      | -1.75078E-03
      | -8.64221E-04
      | 2.23377E-05
      | 9.08896E-04
      | 1.79546E-03
      | 2.68201E-03
      | -2.83738E-03
      | -1.88414E-03
      | -9.30902E-04
      | 2.23377E-05
      | 9.75577E-04
      | 1.92882E-03
      | 2.88206E-03
      | -2.63786E-03
      | -1.74504E-03
      | -8.52211E-04
      | 4.06140E-05
      | 9.33439E-04
      | 1.82626E-03
      | 2.71909E-03
      | -2.63728E-03
      | -1.74465E-03
      | -8.52017E-04
      | 4.06140E-05
      | 9.33245E-04
      | 1.82588E-03
      | 2.71851E-03
      | -2.86138E-03
      | -1.89405E-03
      | -9.26716E-04
      | 4.06140E-05
      | 1.00794E-03
      | 1.97527E-03
      | 2.94260E-03
      | -0.002723494
      | -0.001792522
      | -0.000861549
      | 6.9423E-05
      | 0.001000396
      | 0.001931368
      | 0.002862341
      | -0.002736476
      | -0.001798489
      | -0.000860502
      | 6.9423E-05
      | 0.001015473
      | 0.00195346
      | 0.002891447
      | -0.002765582
      | -0.00182058
      | -0.000875579
      | 6.9423E-05
      | 0.001014425
      | 0.001959426
      | 0.002904428],[7,3,4])
      BreakpointsForDimension3=|
      | [-35.0624 -18.3724 -15.3724 -13.8724
      | ]
      settings: InputPortMap=u0,u1,u2
  Mdxi : Subsystem
  Mqq2 : Lookup_n-D  NumberOfTableDimensions=1  BreakpointsForDimension1=|  Table=|  InternalRulePriority=Speed  RndMeth=Simplest
      BreakpointsForDimension1=|
      | [-0.02
      | -0.015
      | -0.012958963
      | -0.009719222
      | -0.006479482
      | -0.003239741
      | -0.00161987
      | -0.000647948
      | 0.000647948
      | 0.00161987
      | 0.003239741
      | 0.006479482
      | 0.009719222
      | 0.012958963
      | 0.015
      | 0.02
      | ]
      Table=|
      | [-2.2571E-03
      | -2.3029E-03
      | -2.0965E-03
      | -2.0229E-03
      | -2.1546E-03
      | -1.4789E-03
      | -1.5664E-03
      | -1.4544E-03
      | -1.4705E-03
      | -1.4942E-03
      | -1.8790E-03
      | -1.8821E-03
      | -2.1009E-03
      | -2.0521E-03
      | -2.1685E-03
      | -2.0822E-03
      | ]
  Mwq : Lookup_n-D  NumberOfTableDimensions=1  BreakpointsForDimension1=|  Table=|  InternalRulePriority=Speed  RndMeth=Simplest
      BreakpointsForDimension1=|
      | [-0.0015
      | -0.0012
      | -0.0009
      | -0.0006
      | -0.0003
      | -0.0001
      | 0.0001
      | 0.0003
      | 0.0006
      | 0.0009
      | 0.0012
      | 0.0015]
      Table=|
      | [-1.3011E-02
      | -1.6962E-02
      | -2.0682E-02
      | -3.1419E-02
      | -6.4407E-02
      | -1.9322E-01
      | 1.9322E-01
      | 6.4378E-02
      | 3.1944E-02
      | 2.1072E-02
      | 1.6415E-02
      | 1.3407E-02]
  My : MATLAB Function  TreatAsAtomicUnit=on
  Product5 : Product
  Saturation2 : Saturate  UpperLimit=0.0015  LowerLimit=-0.0015
  Saturation3 : Saturate  UpperLimit=0.02  LowerLimit=-0.02
  Saturation4 : Saturate  UpperLimit=-13.8724  LowerLimit=-35.0624
  Selector1 : Selector  InputPortWidth=6  IndexOptions=Index vector (dialog)  Indices=5  OutputSizes=1
  Selector10 : Selector  InputPortWidth=6  IndexOptions=Index vector (dialog)  Indices=1  OutputSizes=1
  Selector2 : Selector  InputPortWidth=6  IndexOptions=Index vector (dialog)  Indices=3  OutputSizes=1
  Selector4 : Selector  InputPortWidth=6  IndexOptions=Index vector (dialog)  Indices=5  OutputSizes=1
  Selector8 : Selector  InputPortWidth=6  IndexOptions=Index vector (dialog)  Indices=3  OutputSizes=1
  M : Outport
  wires:
  Gain1/1 -> My/12(MdXi)
  My/4(Mprop) -> [M_Prop]
  My/6(MY_hyd) -> [M_Hyd]
  My/5(M_hull) -> [M_Hull]
  My/2(MYApp) -> [M_App]
  Selector1/1 -> My/14(BFM)
  BFM/1 -> Selector1/1
  Gain/1 -> My/7(Muvw)
  Saturation4/1 -> M_uvwa/3, Mdxi/2(z)  "z"
  My/3(MYStat) -> [M_stat]
  Bv/1 -> My/2(Bv), Selector4/1, Selector8/1, Selector10/1
  Bx/1 -> My/1(Bx), Selector2/1
  Selector10/1 -> M'prop/1, M_uvwa/2  "speed"
  Ba/1 -> My/3(Ba)
  M'prop/1 -> My/6("Mprop ")
  UeSP/1 -> My/9(UeSP)
  Selector4/1 -> Saturation3/1, Abs/1
  Alpha/1 -> M_uvwa/1  "AOA"
  Umag/1 -> My/8(Umag)
  dLCG/1 -> My/10(dLCG)
  dmass/1 -> My/11(dmass)
  dX/1 -> Mdxi/1(dX)
  Mqq2/1 -> My/4(Mqq)
  Mwq/1 -> My/5(Mwq)
  Product5/1 -> Saturation2/1
  Selector8/1 -> Product5/2
  Abs/1 -> Product5/1
  Saturation2/1 -> Mwq/1
  Saturation3/1 -> Mqq2/1
  My/1(MY) -> [M_Total], M/1
  Mdxi/1(MdX) -> Gain1/1
  Mvm/1 -> [Mvm], My/13(Mvm)
  Selector2/1 -> Saturation4/1
  M_uvwa/1 -> Gain/1
